simulink model "BasicAffineLPVmodel_mdl"  (R2018b)
settings: Solver=VariableStepAuto  StartTime=0.0  StopTime=5  MaxStep=0.01  RelTol=1e-3  EnableMultiTasking=on
libraries: lpvlibrary x2, simulink x1
settings Model: Creator=Fernando  LastModifiedBy=ferna
settings OptimizationCC: LifeSpan=inf
settings DebuggingCC: SFUnexpectedBacktrackingDiag=warning  SFNoUnconditionalDefaultTransitionDiag=warning
settings SFSimCC: SimUseLocalCustomCode=off
settings RTWCC: RTWUseLocalCustomCode=off
settings CodeAppCC: StateflowObjectComments=on
settings GRTTargetCC: TargetLangStandard=C89/C90 (ANSI)  GeneratePreprocessorConditionals=Disable all
settings ConfigComp: CovMetricSettings=dw  CovHtmlReporting=on  CovSaveCumulativeToWorkspaceVar=on  CovSaveSingleToWorkspaceVar=on  CovExternalEMLEnable=off

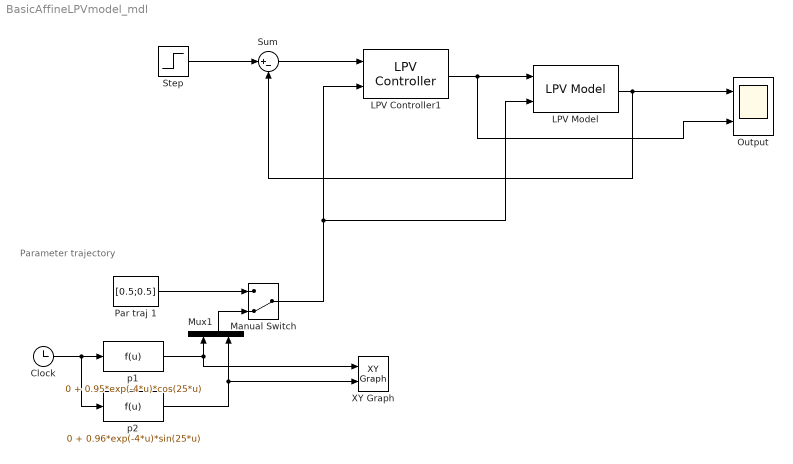
== system BasicAffineLPVmodel_mdl ==
  note: Parameter trajectory
  Clock : Clock
  LPV Controller1 : lpvlibrary/LPV Controller  pdK=pdKp1  x0=0
      settings: SourceProductName=LPV Toolbox
  LPV Model : lpvlibrary/LPV Model  pdG=pdG  x0=0
      settings: SourceProductName=LPV Toolbox
  Manual Switch : ManualSwitch  CurrentSetting=0
  Mux1 : Mux  Inputs=2
  Output : Scope  NumInputPorts=2
  Par traj 1 : Constant  Value=[0.5;0.5]
  Step : Step  Time=0.2  SampleTime=0
  Sum : Sum  Inputs=|+-
  XY Graph : simulink/Sinks/XY Graph  xmin=-1  xmax=1  ymin=-1  ymax=1  st=-1
  p1 : Fcn  Expr=0 + 0.95*exp(-4*u)*cos(25*u)
  p2 : Fcn  Expr=0 + 0.96*exp(-4*u)*sin(25*u)
  wires:
  Clock/1 -> p2/1, p1/1
  p1/1 -> XY Graph/1, Mux1/1
  p2/1 -> Mux1/2, XY Graph/2
  Mux1/1 -> Manual Switch/2
  Par traj 1/1 -> Manual Switch/1
  LPV Controller1/1 -> LPV Model/1, Output/2
  Sum/1 -> LPV Controller1/1
  LPV Model/1 -> Output/1, Sum/2
  Step/1 -> Sum/1
  Manual Switch/1 -> LPV Controller1/2, LPV Model/2
